simulink model "TSR_Scenario_002_cs"  (R2014b)
settings: Solver=ode5  SolverMode=SingleTasking  StartTime=0.0  StopTime=inf  FixedStep=1/100  RelTol=1e-3
PreLoadFcn:
  | mbxruntime.callbacks.PreLoadFcn(bdroot);
  | check_NUTS_defined;
  | 
  | assignin('base',['model_closed_' bdroot],false);
  | 
  | addpath('../includes_TSR/includes_TSR');
  | 
  | switch version('-release')
  | case {'2010a', '2010b', '2011a'}
  | addpath('../includes_TSR/ML2010b');
  | otherwise
  | addpath('../includes_TSR/ML2011b');
  | end
PostLoadFcn:
  | mbxruntime.callbacks.PostLoadFcn(bdroot);
InitFcn:
  | mbxruntime.callbacks.InitFcn(bdroot);;
  | 
  | addpath('..\includes_TSR');
StartFcn:
  | mbxruntime.callbacks.StartFcn(bdroot);
StopFcn:
  | mbxruntime.callbacks.StopFcn(bdroot);
model workspace: external: MAT-File .\TSR_Scenario_002_cs_hws.mat (data not in the file)
undefined symbols (not defined in the file or in its folder): InitImageOutputDir, mbxruntime, OrientationPitch, OrientationRoll, PositionX, PositionY, PositionZ, tabledata, warningInitialVelocity, x0
undefined symbols (not defined in the file): SteeringColumn, SteeringWheel, TSR_Scenario_002_cs_003e47b1b59594b6, TSR_Scenario_002_cs_023e87a31011dc74, TSR_Scenario_002_cs_048cb8409c90d9c6, TSR_Scenario_002_cs_106a0284aafa53e6, TSR_Scenario_002_cs_195b368d22a7f172, TSR_Scenario_002_cs_1e339fa5d680f213, TSR_Scenario_002_cs_26196a9fb104f950, TSR_Scenario_002_cs_261a709f6f453598, TSR_Scenario_002_cs_2ac3337370d0049d, TSR_Scenario_002_cs_2dc51e6a68b01b00, TSR_Scenario_002_cs_3460ff54d38ab2e2, TSR_Scenario_002_cs_42ea7d6e56bd6005, TSR_Scenario_002_cs_4dd419d6d2b56fc2, TSR_Scenario_002_cs_5316a21de09dff2f, TSR_Scenario_002_cs_538caacf3455966d, TSR_Scenario_002_cs_5b2cfdbcfc80811f, TSR_Scenario_002_cs_5ce0eafbb7a2dce7, TSR_Scenario_002_cs_62cdbf45c6f8824a, TSR_Scenario_002_cs_6bebc368eedff0bc, TSR_Scenario_002_cs_6d26481da4ed7e29, TSR_Scenario_002_cs_70c7e369ce6550e0, TSR_Scenario_002_cs_7a63051a1f311451, TSR_Scenario_002_cs_7d7dc8405f613c6d, TSR_Scenario_002_cs_7f65e296173485e8, TSR_Scenario_002_cs_87183cf6ff7bb4b6, TSR_Scenario_002_cs_8921b0da7ab80865, TSR_Scenario_002_cs_9495ce3a76763d1f, TSR_Scenario_002_cs_a679806a2fdc8099, TSR_Scenario_002_cs_Actros_1860_1_Path_pathUniqueID, TSR_Scenario_002_cs_Actros_2541_1_Path_pathUniqueID, TSR_Scenario_002_cs_Actros_2541_3_Path_pathUniqueID, TSR_Scenario_002_cs_Actros_2541_4_Path_pathUniqueID, TSR_Scenario_002_cs_adf24c93a9de8a4e, TSR_Scenario_002_cs_Audi_A8_1_Dynamics_Simple_initialPitch, TSR_Scenario_002_cs_Audi_A8_1_Dynamics_Simple_initialRoll, TSR_Scenario_002_cs_Audi_A8_1_Dynamics_Simple_initialX, TSR_Scenario_002_cs_Audi_A8_1_Dynamics_Simple_initialY, TSR_Scenario_002_cs_Audi_A8_1_Dynamics_Simple_initialYaw, TSR_Scenario_002_cs_Audi_A8_1_Dynamics_Simple_initialZ, TSR_Scenario_002_cs_b136c6ccb55f77db, TSR_Scenario_002_cs_ba4f809714c282b7, TSR_Scenario_002_cs_BMW_X5_1_Path_pathUniqueID, TSR_Scenario_002_cs_BMW_X5_1_SpeedProfile_speedProfileUniqueID, TSR_Scenario_002_cs_BMW_X5_2_Path_pathUniqueID, TSR_Scenario_002_cs_BMW_X5_2_SpeedProfile_speedProfileUniqueID, TSR_Scenario_002_cs_Citroen_C3_1_Path_pathUniqueID, TSR_Scenario_002_cs_Citroen_C3_2_Path_pathUniqueID, TSR_Scenario_002_cs_d8f275339b7082cf, TSR_Scenario_002_cs_Daf_95_1_Path_pathUniqueID, TSR_Scenario_002_cs_Daf_95_1_SpeedProfile_speedProfileUniqueID, TSR_Scenario_002_cs_dc019741510ce2f2, TSR_Scenario_002_cs_fdbc8aabe460b27c, TSR_Scenario_002_cs_Fiat_Bravo_1_Path_pathUniqueID, TSR_Scenario_002_cs_Ford_Fiesta_1_Path_pathUniqueID, TSR_Scenario_002_cs_Honda_Pan_European_1_Path_pathUniqueID, TSR_Scenario_002_cs_Mazda_RX8_1_Path_pathUniqueID, TSR_Scenario_002_cs_Nissan_Cabstar_1_Path_pathUniqueID, TSR_Scenario_002_cs_Nissan_Cabstar_2_Path_pathUniqueID ... (+9)
libraries: simulink_extras x82, simulink x23, PreScanSimulinkLibrary x11
(part 20 of 39)

== system TSR_Scenario_002_cs/Fiat_Bravo_1/SELF_Demux ==
  SELF : Inport  OutDataTypeStr=Bus: PRESCAN_SELFSENSORDATA
  Bus Selector : BusSelector  OutputSignals=PositionX,PositionY,PositionZ,OrientationRoll,OrientationPitch,OrientationYaw,Velocity,Yaw_rate,Lat,Long,Alt
  Demux2 : Demux  Outputs=3
  Gain : Gain  Gain=180/pi
  Gain1 : Gain  Gain=180/pi
  Vector Concatenate1 : Concatenate  NumInputs=3
  compas converter : Subsystem
  x [m] : Outport
  y [m] : Outport  Port=2
  z [m] : Outport  Port=3
  rotx [deg] : Outport  Port=4
  roty [deg] : Outport  Port=5
  rotz [deg] : Outport  Port=6
  GPS lat [deg] : Outport  Port=7
  GPS long [deg] : Outport  Port=8
  GPS alt [m] : Outport  Port=9
  velocity [m/s] : Outport  Port=10
  heading [deg] : Outport  Port=11
  yaw rate [deg/s] : Outport  Port=12
  wires:
  Bus Selector/11 -> GPS alt [m]/1  "<Alt>"
  Bus Selector/10 -> GPS long [deg]/1  "<Long>"
  Bus Selector/9 -> GPS lat [deg]/1  "<Lat>"
  Bus Selector/8 -> Gain1/1  "<Yaw_rate>"
  Bus Selector/7 -> velocity [m/s]/1  "<Velocity>"
  Bus Selector/6 -> compas converter/1(rotz [rad]), Vector Concatenate1/3  "<OrientationYaw>"
  Bus Selector/5 -> Vector Concatenate1/2  "<OrientationPitch>"
  Bus Selector/4 -> Vector Concatenate1/1  "<OrientationRoll>"
  Vector Concatenate1/1 -> Gain/1
  Bus Selector/3 -> z [m]/1  "<PositionZ>"
  Bus Selector/2 -> y [m]/1  "<PositionY>"
  Bus Selector/1 -> x [m]/1  "<PositionX>"
  SELF/1 -> Bus Selector/1
  Gain/1 -> Demux2/1
  Demux2/1 -> rotx [deg]/1
  Demux2/2 -> roty [deg]/1
  Demux2/3 -> rotz [deg]/1
  compas converter/1(heading [deg]) -> heading [deg]/1
  Gain1/1 -> yaw rate [deg/s]/1

== system TSR_Scenario_002_cs/Fiat_Bravo_1/SteeringColumn_pivot_Mux ==
  X [m] : Inport
  Y [m] : Inport  Port=2
  Z [m] : Inport  Port=3
  Roll [rad] : Inport  Port=4
  Pitch [rad] : Inport  Port=5
  Yaw [rad] : Inport  Port=6
  Bus Creator : BusCreator  Inputs=3  OutDataTypeStr=Bus: PRESCAN_XYZ_DATA
  Bus Creator1 : BusCreator  Inputs=3  OutDataTypeStr=Bus: PRESCAN_RPY_DATA
  Bus Creator2 : BusCreator  Inputs=2  OutDataTypeStr=Bus: PRESCAN_POSE_DATA
  Joint : Outport
  wires:
  Yaw [rad]/1 -> Bus Creator1/3  "Yaw"
  Bus Creator1/1 -> Bus Creator2/2  "ORIENTATION"
  Bus Creator/1 -> Bus Creator2/1  "POSITION"
  X [m]/1 -> Bus Creator/1  "X"
  Y [m]/1 -> Bus Creator/2  "Y"
  Z [m]/1 -> Bus Creator/3  "Z"
  Bus Creator2/1 -> Joint/1
  Roll [rad]/1 -> Bus Creator1/1  "Roll"
  Pitch [rad]/1 -> Bus Creator1/2  "Pitch"

== system TSR_Scenario_002_cs/Fiat_Bravo_1/SteeringWheel_pivot_Mux ==
  X [m] : Inport
  Y [m] : Inport  Port=2
  Z [m] : Inport  Port=3
  Roll [rad] : Inport  Port=4
  Pitch [rad] : Inport  Port=5
  Yaw [rad] : Inport  Port=6
  Bus Creator : BusCreator  Inputs=3  OutDataTypeStr=Bus: PRESCAN_XYZ_DATA
  Bus Creator1 : BusCreator  Inputs=3  OutDataTypeStr=Bus: PRESCAN_RPY_DATA
  Bus Creator2 : BusCreator  Inputs=2  OutDataTypeStr=Bus: PRESCAN_POSE_DATA
  Joint : Outport
  wires:
  Yaw [rad]/1 -> Bus Creator1/3  "Yaw"
  Bus Creator1/1 -> Bus Creator2/2  "ORIENTATION"
  Bus Creator/1 -> Bus Creator2/1  "POSITION"
  X [m]/1 -> Bus Creator/1  "X"
  Y [m]/1 -> Bus Creator/2  "Y"
  Z [m]/1 -> Bus Creator/3  "Z"
  Bus Creator2/1 -> Joint/1
  Roll [rad]/1 -> Bus Creator1/1  "Roll"
  Pitch [rad]/1 -> Bus Creator1/2  "Pitch"

== system TSR_Scenario_002_cs/Fiat_Bravo_1/WheelDisplacement_Mux ==
  Steering Angle Front [rad] : Inport  Tag=inport/JointGroup  SampleTime=1/100  BusOutputAsStruct=on
  Steering Angle Rear [rad] : Inport  Tag=inport/JointGroup  Port=2  SampleTime=1/100  BusOutputAsStruct=on
  Rotation [rad] : Inport  Tag=inport/JointGroup  Port=3  SampleTime=1/100  BusOutputAsStruct=on
  zDisp FL [m] : Inport  Tag=inport/JointGroup  Port=4  SampleTime=1/100  BusOutputAsStruct=on
  zDisp FR [m] : Inport  Tag=inport/JointGroup  Port=5  SampleTime=1/100  BusOutputAsStruct=on
  zDisp RL [m] : Inport  Tag=inport/JointGroup  Port=6  SampleTime=1/100  BusOutputAsStruct=on
  zDisp RR [m] : Inport  Tag=inport/JointGroup  Port=7  SampleTime=1/100  BusOutputAsStruct=on
  Ground_{1..12} (12 alike) : Ground
  WheelL0_Mux : Subsystem  Tag=mux/Joint  mask(PreScan Mux Block){DisplayName=WheelL0}
      mask prompts: DisplayName "Display Name"
      mask help:
      | This block simulates a generic joint used for generic models. This joint can be enabled/disabled from the GUI.
      |
      | For more information, please click Help.
      settings: DeleteFcn=PreScanBlockDeleteFcn;
      mask Help: eval('openHelp(254)')
  WheelL1_Mux : Subsystem  Tag=mux/Joint  mask(PreScan Mux Block){DisplayName=WheelL1}
      mask prompts: DisplayName "Display Name"
      mask help:
      | This block simulates a generic joint used for generic models. This joint can be enabled/disabled from the GUI.
      |
      | For more information, please click Help.
      settings: DeleteFcn=PreScanBlockDeleteFcn;
      mask Help: eval('openHelp(254)')
  WheelR0_Mux : Subsystem  Tag=mux/Joint  mask(PreScan Mux Block){DisplayName=WheelR0}
      mask prompts: DisplayName "Display Name"
      mask help:
      | This block simulates a generic joint used for generic models. This joint can be enabled/disabled from the GUI.
      |
      | For more information, please click Help.
      settings: DeleteFcn=PreScanBlockDeleteFcn;
      mask Help: eval('openHelp(254)')
  WheelR1_Mux : Subsystem  Tag=mux/Joint  mask(PreScan Mux Block){DisplayName=WheelR1}
      mask prompts: DisplayName "Display Name"
      mask help:
      | This block simulates a generic joint used for generic models. This joint can be enabled/disabled from the GUI.
      |
      | For more information, please click Help.
      settings: DeleteFcn=PreScanBlockDeleteFcn;
      mask Help: eval('openHelp(254)')
  WheelL0_Fiat_Bravo_1 : Outport  Tag=outport/JointActuator  OutDataTypeStr=Bus: PRESCAN_POSE_DATA  SampleTime=1/100
  WheelL1_Fiat_Bravo_1 : Outport  Tag=outport/JointActuator  Port=2  OutDataTypeStr=Bus: PRESCAN_POSE_DATA  SampleTime=1/100
  WheelR0_Fiat_Bravo_1 : Outport  Tag=outport/JointActuator  Port=3  OutDataTypeStr=Bus: PRESCAN_POSE_DATA  SampleTime=1/100
  WheelR1_Fiat_Bravo_1 : Outport  Tag=outport/JointActuator  Port=4  OutDataTypeStr=Bus: PRESCAN_POSE_DATA  SampleTime=1/100
  wires:
  WheelL0_Mux/1(Joint) -> WheelL0_Fiat_Bravo_1/1
  WheelL1_Mux/1(Joint) -> WheelL1_Fiat_Bravo_1/1
  WheelR0_Mux/1(Joint) -> WheelR0_Fiat_Bravo_1/1
  WheelR1_Mux/1(Joint) -> WheelR1_Fiat_Bravo_1/1
  Steering Angle Front [rad]/1 -> WheelR0_Mux/6(Yaw [rad]), WheelL0_Mux/6(Yaw [rad])
  Steering Angle Rear [rad]/1 -> WheelR1_Mux/6(Yaw [rad]), WheelL1_Mux/6(Yaw [rad])
  Rotation [rad]/1 -> WheelR0_Mux/5(Pitch [rad]), WheelL0_Mux/5(Pitch [rad]), WheelR1_Mux/5(Pitch [rad]), WheelL1_Mux/5(Pitch [rad])
  zDisp FL [m]/1 -> WheelL0_Mux/3(Z [m])
  zDisp FR [m]/1 -> WheelR0_Mux/3(Z [m])
  zDisp RL [m]/1 -> WheelL1_Mux/3(Z [m])
  zDisp RR [m]/1 -> WheelR1_Mux/3(Z [m])
  Ground_1/1 -> WheelL0_Mux/1(X [m])
  Ground_2/1 -> WheelL0_Mux/2(Y [m])
  Ground_3/1 -> WheelL0_Mux/4(Roll [rad])
  Ground_4/1 -> WheelL1_Mux/1(X [m])
  Ground_5/1 -> WheelL1_Mux/2(Y [m])
  Ground_6/1 -> WheelL1_Mux/4(Roll [rad])
  Ground_7/1 -> WheelR0_Mux/1(X [m])
  Ground_8/1 -> WheelR0_Mux/2(Y [m])
  Ground_9/1 -> WheelR0_Mux/4(Roll [rad])
  Ground_10/1 -> WheelR1_Mux/1(X [m])
  Ground_11/1 -> WheelR1_Mux/2(Y [m])
  Ground_12/1 -> WheelR1_Mux/4(Roll [rad])

== system TSR_Scenario_002_cs/Ford_Fiesta_1/SELF_Demux ==
  SELF : Inport  OutDataTypeStr=Bus: PRESCAN_SELFSENSORDATA
  Bus Selector : BusSelector  OutputSignals=PositionX,PositionY,PositionZ,OrientationRoll,OrientationPitch,OrientationYaw,Velocity,Yaw_rate,Lat,Long,Alt
  Demux2 : Demux  Outputs=3
  Gain : Gain  Gain=180/pi
  Gain1 : Gain  Gain=180/pi
  Vector Concatenate1 : Concatenate  NumInputs=3
  compas converter : Subsystem
  x [m] : Outport
  y [m] : Outport  Port=2
  z [m] : Outport  Port=3
  rotx [deg] : Outport  Port=4
  roty [deg] : Outport  Port=5
  rotz [deg] : Outport  Port=6
  GPS lat [deg] : Outport  Port=7
  GPS long [deg] : Outport  Port=8
  GPS alt [m] : Outport  Port=9
  velocity [m/s] : Outport  Port=10
  heading [deg] : Outport  Port=11
  yaw rate [deg/s] : Outport  Port=12
  wires:
  Bus Selector/11 -> GPS alt [m]/1  "<Alt>"
  Bus Selector/10 -> GPS long [deg]/1  "<Long>"
  Bus Selector/9 -> GPS lat [deg]/1  "<Lat>"
  Bus Selector/8 -> Gain1/1  "<Yaw_rate>"
  Bus Selector/7 -> velocity [m/s]/1  "<Velocity>"
  Bus Selector/6 -> compas converter/1(rotz [rad]), Vector Concatenate1/3  "<OrientationYaw>"
  Bus Selector/5 -> Vector Concatenate1/2  "<OrientationPitch>"
  Bus Selector/4 -> Vector Concatenate1/1  "<OrientationRoll>"
  Vector Concatenate1/1 -> Gain/1
  Bus Selector/3 -> z [m]/1  "<PositionZ>"
  Bus Selector/2 -> y [m]/1  "<PositionY>"
  Bus Selector/1 -> x [m]/1  "<PositionX>"
  SELF/1 -> Bus Selector/1
  Gain/1 -> Demux2/1
  Demux2/1 -> rotx [deg]/1
  Demux2/2 -> roty [deg]/1
  Demux2/3 -> rotz [deg]/1
  compas converter/1(heading [deg]) -> heading [deg]/1
  Gain1/1 -> yaw rate [deg/s]/1

== system TSR_Scenario_002_cs/HighwayOverhang_1/VISUMatrixSignLights_Mux ==
  MatrixSign_1 : Inport  Tag=inport/MatrixSign_1  PortDimensions=4  SampleTime=1/100  BusOutputAsStruct=on
  MatrixSign_43 : Inport  Tag=inport/MatrixSign_43  Port=2  PortDimensions=4  SampleTime=1/100  BusOutputAsStruct=on
  MuxVisuLights : Mux  Inputs=2
  VISUMatrixSignLights_HighwayOverhang_1 : Outport  Tag=outport/VisuMatrixSignLights  SampleTime=1/100
  wires:
  MuxVisuLights/1 -> VISUMatrixSignLights_HighwayOverhang_1/1
  MatrixSign_1/1 -> MuxVisuLights/1
  MatrixSign_43/1 -> MuxVisuLights/2

== system TSR_Scenario_002_cs/HighwayOverhang_1/VISUMatrixSign_Mux ==
  MatrixSign_1 : Inport
  MatrixSign_43 : Inport  Port=2
  MatrixSign_1_Conversion : DataTypeConversion
  MatrixSign_1_InitialResource : Constant  Value=17
  MatrixSign_1_Switch : Switch  Criteria=u2 ~= 0
  MatrixSign_43_Conversion : DataTypeConversion
  MatrixSign_43_InitialResource : Constant  Value=17
  MatrixSign_43_Switch : Switch  Criteria=u2 ~= 0
  SubMuxMatrixSign : Mux  Inputs=2
  MatrixSigns : Outport
  wires:
  SubMuxMatrixSign/1 -> MatrixSigns/1
  MatrixSign_1/1 -> MatrixSign_1_Switch/1, MatrixSign_1_Switch/2
  MatrixSign_1_InitialResource/1 -> MatrixSign_1_Switch/3
  MatrixSign_1_Switch/1 -> MatrixSign_1_Conversion/1
  MatrixSign_1_Conversion/1 -> SubMuxMatrixSign/1
  MatrixSign_43/1 -> MatrixSign_43_Switch/1, MatrixSign_43_Switch/2
  MatrixSign_43_InitialResource/1 -> MatrixSign_43_Switch/3
  MatrixSign_43_Switch/1 -> MatrixSign_43_Conversion/1
  MatrixSign_43_Conversion/1 -> SubMuxMatrixSign/2

== system TSR_Scenario_002_cs/HighwayOverhang_10/VISUMatrixSignLights_Mux ==
  MatrixSign_17 : Inport  Tag=inport/MatrixSign_17  PortDimensions=4  SampleTime=1/100  BusOutputAsStruct=on
  MatrixSign_18 : Inport  Tag=inport/MatrixSign_18  Port=2  PortDimensions=4  SampleTime=1/100  BusOutputAsStruct=on
  MuxVisuLights : Mux  Inputs=2
  VISUMatrixSignLights_HighwayOverhang_10 : Outport  Tag=outport/VisuMatrixSignLights  SampleTime=1/100
  wires:
  MuxVisuLights/1 -> VISUMatrixSignLights_HighwayOverhang_10/1
  MatrixSign_17/1 -> MuxVisuLights/1
  MatrixSign_18/1 -> MuxVisuLights/2

== system TSR_Scenario_002_cs/HighwayOverhang_10/VISUMatrixSign_Mux ==
  MatrixSign_17 : Inport
  MatrixSign_18 : Inport  Port=2
  MatrixSign_17_Conversion : DataTypeConversion
  MatrixSign_17_InitialResource : Constant
  MatrixSign_17_Switch : Switch  Criteria=u2 ~= 0
  MatrixSign_18_Conversion : DataTypeConversion
  MatrixSign_18_InitialResource : Constant
  MatrixSign_18_Switch : Switch  Criteria=u2 ~= 0
  SubMuxMatrixSign : Mux  Inputs=2
  MatrixSigns : Outport
  wires:
  SubMuxMatrixSign/1 -> MatrixSigns/1
  MatrixSign_17/1 -> MatrixSign_17_Switch/1, MatrixSign_17_Switch/2
  MatrixSign_17_InitialResource/1 -> MatrixSign_17_Switch/3
  MatrixSign_17_Switch/1 -> MatrixSign_17_Conversion/1
  MatrixSign_17_Conversion/1 -> SubMuxMatrixSign/1
  MatrixSign_18/1 -> MatrixSign_18_Switch/1, MatrixSign_18_Switch/2
  MatrixSign_18_InitialResource/1 -> MatrixSign_18_Switch/3
  MatrixSign_18_Switch/1 -> MatrixSign_18_Conversion/1
  MatrixSign_18_Conversion/1 -> SubMuxMatrixSign/2

== system TSR_Scenario_002_cs/HighwayOverhang_11/VISUMatrixSignLights_Mux ==
  MatrixSign_10 : Inport  Tag=inport/MatrixSign_10  PortDimensions=4  SampleTime=1/100  BusOutputAsStruct=on
  MatrixSign_49 : Inport  Tag=inport/MatrixSign_49  Port=2  PortDimensions=4  SampleTime=1/100  BusOutputAsStruct=on
  MuxVisuLights : Mux  Inputs=2
  VISUMatrixSignLights_HighwayOverhang_11 : Outport  Tag=outport/VisuMatrixSignLights  SampleTime=1/100
  wires:
  MuxVisuLights/1 -> VISUMatrixSignLights_HighwayOverhang_11/1
  MatrixSign_10/1 -> MuxVisuLights/1
  MatrixSign_49/1 -> MuxVisuLights/2

== system TSR_Scenario_002_cs/HighwayOverhang_11/VISUMatrixSign_Mux ==
  MatrixSign_10 : Inport
  MatrixSign_49 : Inport  Port=2
  MatrixSign_10_Conversion : DataTypeConversion
  MatrixSign_10_InitialResource : Constant  Value=11
  MatrixSign_10_Switch : Switch  Criteria=u2 ~= 0
  MatrixSign_49_Conversion : DataTypeConversion
  MatrixSign_49_InitialResource : Constant  Value=11
  MatrixSign_49_Switch : Switch  Criteria=u2 ~= 0
  SubMuxMatrixSign : Mux  Inputs=2
  MatrixSigns : Outport
  wires:
  SubMuxMatrixSign/1 -> MatrixSigns/1
  MatrixSign_10/1 -> MatrixSign_10_Switch/1, MatrixSign_10_Switch/2
  MatrixSign_10_InitialResource/1 -> MatrixSign_10_Switch/3
  MatrixSign_10_Switch/1 -> MatrixSign_10_Conversion/1
  MatrixSign_10_Conversion/1 -> SubMuxMatrixSign/1
  MatrixSign_49/1 -> MatrixSign_49_Switch/1, MatrixSign_49_Switch/2
  MatrixSign_49_InitialResource/1 -> MatrixSign_49_Switch/3
  MatrixSign_49_Switch/1 -> MatrixSign_49_Conversion/1
  MatrixSign_49_Conversion/1 -> SubMuxMatrixSign/2

== system TSR_Scenario_002_cs/HighwayOverhang_12/VISUMatrixSignLights_Mux ==
  MatrixSign_21 : Inport  Tag=inport/MatrixSign_21  PortDimensions=4  SampleTime=1/100  BusOutputAsStruct=on
  MatrixSign_22 : Inport  Tag=inport/MatrixSign_22  Port=2  PortDimensions=4  SampleTime=1/100  BusOutputAsStruct=on
  MuxVisuLights : Mux  Inputs=2
  VISUMatrixSignLights_HighwayOverhang_12 : Outport  Tag=outport/VisuMatrixSignLights  SampleTime=1/100
  wires:
  MuxVisuLights/1 -> VISUMatrixSignLights_HighwayOverhang_12/1
  MatrixSign_21/1 -> MuxVisuLights/1
  MatrixSign_22/1 -> MuxVisuLights/2

== system TSR_Scenario_002_cs/HighwayOverhang_12/VISUMatrixSign_Mux ==
  MatrixSign_21 : Inport
  MatrixSign_22 : Inport  Port=2
  MatrixSign_21_Conversion : DataTypeConversion
  MatrixSign_21_InitialResource : Constant
  MatrixSign_21_Switch : Switch  Criteria=u2 ~= 0
  MatrixSign_22_Conversion : DataTypeConversion
  MatrixSign_22_InitialResource : Constant
  MatrixSign_22_Switch : Switch  Criteria=u2 ~= 0
  SubMuxMatrixSign : Mux  Inputs=2
  MatrixSigns : Outport
  wires:
  SubMuxMatrixSign/1 -> MatrixSigns/1
  MatrixSign_21/1 -> MatrixSign_21_Switch/1, MatrixSign_21_Switch/2
  MatrixSign_21_InitialResource/1 -> MatrixSign_21_Switch/3
  MatrixSign_21_Switch/1 -> MatrixSign_21_Conversion/1
  MatrixSign_21_Conversion/1 -> SubMuxMatrixSign/1
  MatrixSign_22/1 -> MatrixSign_22_Switch/1, MatrixSign_22_Switch/2
  MatrixSign_22_InitialResource/1 -> MatrixSign_22_Switch/3
  MatrixSign_22_Switch/1 -> MatrixSign_22_Conversion/1
  MatrixSign_22_Conversion/1 -> SubMuxMatrixSign/2

== system TSR_Scenario_002_cs/HighwayOverhang_13/VISUMatrixSignLights_Mux ==
  MatrixSign_3 : Inport  Tag=inport/MatrixSign_3  PortDimensions=4  SampleTime=1/100  BusOutputAsStruct=on
  MatrixSign_44 : Inport  Tag=inport/MatrixSign_44  Port=2  PortDimensions=4  SampleTime=1/100  BusOutputAsStruct=on
  MuxVisuLights : Mux  Inputs=2
  VISUMatrixSignLights_HighwayOverhang_13 : Outport  Tag=outport/VisuMatrixSignLights  SampleTime=1/100
  wires:
  MuxVisuLights/1 -> VISUMatrixSignLights_HighwayOverhang_13/1
  MatrixSign_3/1 -> MuxVisuLights/1
  MatrixSign_44/1 -> MuxVisuLights/2

== system TSR_Scenario_002_cs/HighwayOverhang_13/VISUMatrixSign_Mux ==
  MatrixSign_3 : Inport
  MatrixSign_44 : Inport  Port=2
  MatrixSign_3_Conversion : DataTypeConversion
  MatrixSign_3_InitialResource : Constant  Value=16
  MatrixSign_3_Switch : Switch  Criteria=u2 ~= 0
  MatrixSign_44_Conversion : DataTypeConversion
  MatrixSign_44_InitialResource : Constant  Value=16
  MatrixSign_44_Switch : Switch  Criteria=u2 ~= 0
  SubMuxMatrixSign : Mux  Inputs=2
  MatrixSigns : Outport
  wires:
  SubMuxMatrixSign/1 -> MatrixSigns/1
  MatrixSign_3/1 -> MatrixSign_3_Switch/1, MatrixSign_3_Switch/2
  MatrixSign_3_InitialResource/1 -> MatrixSign_3_Switch/3
  MatrixSign_3_Switch/1 -> MatrixSign_3_Conversion/1
  MatrixSign_3_Conversion/1 -> SubMuxMatrixSign/1
  MatrixSign_44/1 -> MatrixSign_44_Switch/1, MatrixSign_44_Switch/2
  MatrixSign_44_InitialResource/1 -> MatrixSign_44_Switch/3
  MatrixSign_44_Switch/1 -> MatrixSign_44_Conversion/1
  MatrixSign_44_Conversion/1 -> SubMuxMatrixSign/2

== system TSR_Scenario_002_cs/HighwayOverhang_14/VISUMatrixSignLights_Mux ==
  MatrixSign_27 : Inport  Tag=inport/MatrixSign_27  PortDimensions=4  SampleTime=1/100  BusOutputAsStruct=on
  MatrixSign_28 : Inport  Tag=inport/MatrixSign_28  Port=2  PortDimensions=4  SampleTime=1/100  BusOutputAsStruct=on
  MuxVisuLights : Mux  Inputs=2
  VISUMatrixSignLights_HighwayOverhang_14 : Outport  Tag=outport/VisuMatrixSignLights  SampleTime=1/100
  wires:
  MuxVisuLights/1 -> VISUMatrixSignLights_HighwayOverhang_14/1
  MatrixSign_27/1 -> MuxVisuLights/1
  MatrixSign_28/1 -> MuxVisuLights/2

== system TSR_Scenario_002_cs/HighwayOverhang_14/VISUMatrixSign_Mux ==
  MatrixSign_27 : Inport
  MatrixSign_28 : Inport  Port=2
  MatrixSign_27_Conversion : DataTypeConversion
  MatrixSign_27_InitialResource : Constant
  MatrixSign_27_Switch : Switch  Criteria=u2 ~= 0
  MatrixSign_28_Conversion : DataTypeConversion
  MatrixSign_28_InitialResource : Constant
  MatrixSign_28_Switch : Switch  Criteria=u2 ~= 0
  SubMuxMatrixSign : Mux  Inputs=2
  MatrixSigns : Outport
  wires:
  SubMuxMatrixSign/1 -> MatrixSigns/1
  MatrixSign_27/1 -> MatrixSign_27_Switch/1, MatrixSign_27_Switch/2
  MatrixSign_27_InitialResource/1 -> MatrixSign_27_Switch/3
  MatrixSign_27_Switch/1 -> MatrixSign_27_Conversion/1
  MatrixSign_27_Conversion/1 -> SubMuxMatrixSign/1
  MatrixSign_28/1 -> MatrixSign_28_Switch/1, MatrixSign_28_Switch/2
  MatrixSign_28_InitialResource/1 -> MatrixSign_28_Switch/3
  MatrixSign_28_Switch/1 -> MatrixSign_28_Conversion/1
  MatrixSign_28_Conversion/1 -> SubMuxMatrixSign/2

== system TSR_Scenario_002_cs/HighwayOverhang_15/VISUMatrixSignLights_Mux ==
  MatrixSign_46 : Inport  Tag=inport/MatrixSign_46  PortDimensions=4  SampleTime=1/100  BusOutputAsStruct=on
  MatrixSign_5 : Inport  Tag=inport/MatrixSign_5  Port=2  PortDimensions=4  SampleTime=1/100  BusOutputAsStruct=on
  MuxVisuLights : Mux  Inputs=2
  VISUMatrixSignLights_HighwayOverhang_15 : Outport  Tag=outport/VisuMatrixSignLights  SampleTime=1/100
  wires:
  MuxVisuLights/1 -> VISUMatrixSignLights_HighwayOverhang_15/1
  MatrixSign_46/1 -> MuxVisuLights/1
  MatrixSign_5/1 -> MuxVisuLights/2

== system TSR_Scenario_002_cs/HighwayOverhang_15/VISUMatrixSign_Mux ==
  MatrixSign_5 : Inport
  MatrixSign_46 : Inport  Port=2
  MatrixSign_46_Conversion : DataTypeConversion
  MatrixSign_46_InitialResource : Constant  Value=14
  MatrixSign_46_Switch : Switch  Criteria=u2 ~= 0
  MatrixSign_5_Conversion : DataTypeConversion
  MatrixSign_5_InitialResource : Constant  Value=14
  MatrixSign_5_Switch : Switch  Criteria=u2 ~= 0
  SubMuxMatrixSign : Mux  Inputs=2
  MatrixSigns : Outport
  wires:
  SubMuxMatrixSign/1 -> MatrixSigns/1
  MatrixSign_5/1 -> MatrixSign_5_Switch/1, MatrixSign_5_Switch/2
  MatrixSign_5_InitialResource/1 -> MatrixSign_5_Switch/3
  MatrixSign_5_Switch/1 -> MatrixSign_5_Conversion/1
  MatrixSign_5_Conversion/1 -> SubMuxMatrixSign/1
  MatrixSign_46/1 -> MatrixSign_46_Switch/1, MatrixSign_46_Switch/2
  MatrixSign_46_InitialResource/1 -> MatrixSign_46_Switch/3
  MatrixSign_46_Switch/1 -> MatrixSign_46_Conversion/1
  MatrixSign_46_Conversion/1 -> SubMuxMatrixSign/2

== system TSR_Scenario_002_cs/HighwayOverhang_16/VISUMatrixSignLights_Mux ==
  MatrixSign_29 : Inport  Tag=inport/MatrixSign_29  PortDimensions=4  SampleTime=1/100  BusOutputAsStruct=on
  MatrixSign_30 : Inport  Tag=inport/MatrixSign_30  Port=2  PortDimensions=4  SampleTime=1/100  BusOutputAsStruct=on
  MuxVisuLights : Mux  Inputs=2
  VISUMatrixSignLights_HighwayOverhang_16 : Outport  Tag=outport/VisuMatrixSignLights  SampleTime=1/100
  wires:
  MuxVisuLights/1 -> VISUMatrixSignLights_HighwayOverhang_16/1
  MatrixSign_29/1 -> MuxVisuLights/1
  MatrixSign_30/1 -> MuxVisuLights/2

== system TSR_Scenario_002_cs/HighwayOverhang_16/VISUMatrixSign_Mux ==
  MatrixSign_29 : Inport
  MatrixSign_30 : Inport  Port=2
  MatrixSign_29_Conversion : DataTypeConversion
  MatrixSign_29_InitialResource : Constant
  MatrixSign_29_Switch : Switch  Criteria=u2 ~= 0
  MatrixSign_30_Conversion : DataTypeConversion
  MatrixSign_30_InitialResource : Constant
  MatrixSign_30_Switch : Switch  Criteria=u2 ~= 0
  SubMuxMatrixSign : Mux  Inputs=2
  MatrixSigns : Outport
  wires:
  SubMuxMatrixSign/1 -> MatrixSigns/1
  MatrixSign_29/1 -> MatrixSign_29_Switch/1, MatrixSign_29_Switch/2
  MatrixSign_29_InitialResource/1 -> MatrixSign_29_Switch/3
  MatrixSign_29_Switch/1 -> MatrixSign_29_Conversion/1
  MatrixSign_29_Conversion/1 -> SubMuxMatrixSign/1
  MatrixSign_30/1 -> MatrixSign_30_Switch/1, MatrixSign_30_Switch/2
  MatrixSign_30_InitialResource/1 -> MatrixSign_30_Switch/3
  MatrixSign_30_Switch/1 -> MatrixSign_30_Conversion/1
  MatrixSign_30_Conversion/1 -> SubMuxMatrixSign/2

== system TSR_Scenario_002_cs/HighwayOverhang_17/VISUMatrixSignLights_Mux ==
  MatrixSign_51 : Inport  Tag=inport/MatrixSign_51  PortDimensions=4  SampleTime=1/100  BusOutputAsStruct=on
  MatrixSign_7 : Inport  Tag=inport/MatrixSign_7  Port=2  PortDimensions=4  SampleTime=1/100  BusOutputAsStruct=on
  MuxVisuLights : Mux  Inputs=2
  VISUMatrixSignLights_HighwayOverhang_17 : Outport  Tag=outport/VisuMatrixSignLights  SampleTime=1/100
  wires:
  MuxVisuLights/1 -> VISUMatrixSignLights_HighwayOverhang_17/1
  MatrixSign_51/1 -> MuxVisuLights/1
  MatrixSign_7/1 -> MuxVisuLights/2

== system TSR_Scenario_002_cs/HighwayOverhang_17/VISUMatrixSign_Mux ==
  MatrixSign_7 : Inport
  MatrixSign_51 : Inport  Port=2
  MatrixSign_51_Conversion : DataTypeConversion
  MatrixSign_51_InitialResource : Constant  Value=9
  MatrixSign_51_Switch : Switch  Criteria=u2 ~= 0
  MatrixSign_7_Conversion : DataTypeConversion
  MatrixSign_7_InitialResource : Constant  Value=9
  MatrixSign_7_Switch : Switch  Criteria=u2 ~= 0
  SubMuxMatrixSign : Mux  Inputs=2
  MatrixSigns : Outport
  wires:
  SubMuxMatrixSign/1 -> MatrixSigns/1
  MatrixSign_7/1 -> MatrixSign_7_Switch/1, MatrixSign_7_Switch/2
  MatrixSign_7_InitialResource/1 -> MatrixSign_7_Switch/3
  MatrixSign_7_Switch/1 -> MatrixSign_7_Conversion/1
  MatrixSign_7_Conversion/1 -> SubMuxMatrixSign/1
  MatrixSign_51/1 -> MatrixSign_51_Switch/1, MatrixSign_51_Switch/2
  MatrixSign_51_InitialResource/1 -> MatrixSign_51_Switch/3
  MatrixSign_51_Switch/1 -> MatrixSign_51_Conversion/1
  MatrixSign_51_Conversion/1 -> SubMuxMatrixSign/2

== system TSR_Scenario_002_cs/HighwayOverhang_18/VISUMatrixSignLights_Mux ==
  MatrixSign_31 : Inport  Tag=inport/MatrixSign_31  PortDimensions=4  SampleTime=1/100  BusOutputAsStruct=on
  MatrixSign_32 : Inport  Tag=inport/MatrixSign_32  Port=2  PortDimensions=4  SampleTime=1/100  BusOutputAsStruct=on
  MuxVisuLights : Mux  Inputs=2
  VISUMatrixSignLights_HighwayOverhang_18 : Outport  Tag=outport/VisuMatrixSignLights  SampleTime=1/100
  wires:
  MuxVisuLights/1 -> VISUMatrixSignLights_HighwayOverhang_18/1
  MatrixSign_31/1 -> MuxVisuLights/1
  MatrixSign_32/1 -> MuxVisuLights/2

== system TSR_Scenario_002_cs/HighwayOverhang_18/VISUMatrixSign_Mux ==
  MatrixSign_31 : Inport
  MatrixSign_32 : Inport  Port=2
  MatrixSign_31_Conversion : DataTypeConversion
  MatrixSign_31_InitialResource : Constant
  MatrixSign_31_Switch : Switch  Criteria=u2 ~= 0
  MatrixSign_32_Conversion : DataTypeConversion
  MatrixSign_32_InitialResource : Constant
  MatrixSign_32_Switch : Switch  Criteria=u2 ~= 0
  SubMuxMatrixSign : Mux  Inputs=2
  MatrixSigns : Outport
  wires:
  SubMuxMatrixSign/1 -> MatrixSigns/1
  MatrixSign_31/1 -> MatrixSign_31_Switch/1, MatrixSign_31_Switch/2
  MatrixSign_31_InitialResource/1 -> MatrixSign_31_Switch/3
  MatrixSign_31_Switch/1 -> MatrixSign_31_Conversion/1
  MatrixSign_31_Conversion/1 -> SubMuxMatrixSign/1
  MatrixSign_32/1 -> MatrixSign_32_Switch/1, MatrixSign_32_Switch/2
  MatrixSign_32_InitialResource/1 -> MatrixSign_32_Switch/3
  MatrixSign_32_Switch/1 -> MatrixSign_32_Conversion/1
  MatrixSign_32_Conversion/1 -> SubMuxMatrixSign/2

== system TSR_Scenario_002_cs/HighwayOverhang_19/VISUMatrixSignLights_Mux ==
  MatrixSign_52 : Inport  Tag=inport/MatrixSign_52  PortDimensions=4  SampleTime=1/100  BusOutputAsStruct=on
  MatrixSign_9 : Inport  Tag=inport/MatrixSign_9  Port=2  PortDimensions=4  SampleTime=1/100  BusOutputAsStruct=on
  MuxVisuLights : Mux  Inputs=2
  VISUMatrixSignLights_HighwayOverhang_19 : Outport  Tag=outport/VisuMatrixSignLights  SampleTime=1/100
  wires:
  MuxVisuLights/1 -> VISUMatrixSignLights_HighwayOverhang_19/1
  MatrixSign_52/1 -> MuxVisuLights/1
  MatrixSign_9/1 -> MuxVisuLights/2

== system TSR_Scenario_002_cs/HighwayOverhang_19/VISUMatrixSign_Mux ==
  MatrixSign_9 : Inport
  MatrixSign_52 : Inport  Port=2
  MatrixSign_52_Conversion : DataTypeConversion
  MatrixSign_52_InitialResource : Constant  Value=8
  MatrixSign_52_Switch : Switch  Criteria=u2 ~= 0
  MatrixSign_9_Conversion : DataTypeConversion
  MatrixSign_9_InitialResource : Constant  Value=8
  MatrixSign_9_Switch : Switch  Criteria=u2 ~= 0
  SubMuxMatrixSign : Mux  Inputs=2
  MatrixSigns : Outport
  wires:
  SubMuxMatrixSign/1 -> MatrixSigns/1
  MatrixSign_9/1 -> MatrixSign_9_Switch/1, MatrixSign_9_Switch/2
  MatrixSign_9_InitialResource/1 -> MatrixSign_9_Switch/3
  MatrixSign_9_Switch/1 -> MatrixSign_9_Conversion/1
  MatrixSign_9_Conversion/1 -> SubMuxMatrixSign/1
  MatrixSign_52/1 -> MatrixSign_52_Switch/1, MatrixSign_52_Switch/2
  MatrixSign_52_InitialResource/1 -> MatrixSign_52_Switch/3
  MatrixSign_52_Switch/1 -> MatrixSign_52_Conversion/1
  MatrixSign_52_Conversion/1 -> SubMuxMatrixSign/2

== system TSR_Scenario_002_cs/HighwayOverhang_2/VISUMatrixSignLights_Mux ==
  MatrixSign_14 : Inport  Tag=inport/MatrixSign_14  PortDimensions=4  SampleTime=1/100  BusOutputAsStruct=on
  MatrixSign_2 : Inport  Tag=inport/MatrixSign_2  Port=2  PortDimensions=4  SampleTime=1/100  BusOutputAsStruct=on
  MuxVisuLights : Mux  Inputs=2
  VISUMatrixSignLights_HighwayOverhang_2 : Outport  Tag=outport/VisuMatrixSignLights  SampleTime=1/100
  wires:
  MuxVisuLights/1 -> VISUMatrixSignLights_HighwayOverhang_2/1
  MatrixSign_14/1 -> MuxVisuLights/1
  MatrixSign_2/1 -> MuxVisuLights/2

== system TSR_Scenario_002_cs/HighwayOverhang_2/VISUMatrixSign_Mux ==
  MatrixSign_14 : Inport
  MatrixSign_2 : Inport  Port=2
  MatrixSign_14_Conversion : DataTypeConversion
  MatrixSign_14_InitialResource : Constant
  MatrixSign_14_Switch : Switch  Criteria=u2 ~= 0
  MatrixSign_2_Conversion : DataTypeConversion
  MatrixSign_2_InitialResource : Constant
  MatrixSign_2_Switch : Switch  Criteria=u2 ~= 0
  SubMuxMatrixSign : Mux  Inputs=2
  MatrixSigns : Outport
  wires:
  SubMuxMatrixSign/1 -> MatrixSigns/1
  MatrixSign_14/1 -> MatrixSign_14_Switch/1, MatrixSign_14_Switch/2
  MatrixSign_14_InitialResource/1 -> MatrixSign_14_Switch/3
  MatrixSign_14_Switch/1 -> MatrixSign_14_Conversion/1
  MatrixSign_14_Conversion/1 -> SubMuxMatrixSign/1
  MatrixSign_2/1 -> MatrixSign_2_Switch/1, MatrixSign_2_Switch/2
  MatrixSign_2_InitialResource/1 -> MatrixSign_2_Switch/3
  MatrixSign_2_Switch/1 -> MatrixSign_2_Conversion/1
  MatrixSign_2_Conversion/1 -> SubMuxMatrixSign/2

== system TSR_Scenario_002_cs/HighwayOverhang_20/VISUMatrixSignLights_Mux ==
  MatrixSign_33 : Inport  Tag=inport/MatrixSign_33  PortDimensions=4  SampleTime=1/100  BusOutputAsStruct=on
  MatrixSign_34 : Inport  Tag=inport/MatrixSign_34  Port=2  PortDimensions=4  SampleTime=1/100  BusOutputAsStruct=on
  MuxVisuLights : Mux  Inputs=2
  VISUMatrixSignLights_HighwayOverhang_20 : Outport  Tag=outport/VisuMatrixSignLights  SampleTime=1/100
  wires:
  MuxVisuLights/1 -> VISUMatrixSignLights_HighwayOverhang_20/1
  MatrixSign_33/1 -> MuxVisuLights/1
  MatrixSign_34/1 -> MuxVisuLights/2

== system TSR_Scenario_002_cs/HighwayOverhang_20/VISUMatrixSign_Mux ==
  MatrixSign_33 : Inport
  MatrixSign_34 : Inport  Port=2
  MatrixSign_33_Conversion : DataTypeConversion
  MatrixSign_33_InitialResource : Constant
  MatrixSign_33_Switch : Switch  Criteria=u2 ~= 0
  MatrixSign_34_Conversion : DataTypeConversion
  MatrixSign_34_InitialResource : Constant
  MatrixSign_34_Switch : Switch  Criteria=u2 ~= 0
  SubMuxMatrixSign : Mux  Inputs=2
  MatrixSigns : Outport
  wires:
  SubMuxMatrixSign/1 -> MatrixSigns/1
  MatrixSign_33/1 -> MatrixSign_33_Switch/1, MatrixSign_33_Switch/2
  MatrixSign_33_InitialResource/1 -> MatrixSign_33_Switch/3
  MatrixSign_33_Switch/1 -> MatrixSign_33_Conversion/1
  MatrixSign_33_Conversion/1 -> SubMuxMatrixSign/1
  MatrixSign_34/1 -> MatrixSign_34_Switch/1, MatrixSign_34_Switch/2
  MatrixSign_34_InitialResource/1 -> MatrixSign_34_Switch/3
  MatrixSign_34_Switch/1 -> MatrixSign_34_Conversion/1
  MatrixSign_34_Conversion/1 -> SubMuxMatrixSign/2

== system TSR_Scenario_002_cs/HighwayOverhang_21/VISUMatrixSignLights_Mux ==
  MatrixSign_11 : Inport  Tag=inport/MatrixSign_11  PortDimensions=4  SampleTime=1/100  BusOutputAsStruct=on
  MatrixSign_53 : Inport  Tag=inport/MatrixSign_53  Port=2  PortDimensions=4  SampleTime=1/100  BusOutputAsStruct=on
  MuxVisuLights : Mux  Inputs=2
  VISUMatrixSignLights_HighwayOverhang_21 : Outport  Tag=outport/VisuMatrixSignLights  SampleTime=1/100
  wires:
  MuxVisuLights/1 -> VISUMatrixSignLights_HighwayOverhang_21/1
  MatrixSign_11/1 -> MuxVisuLights/1
  MatrixSign_53/1 -> MuxVisuLights/2

== system TSR_Scenario_002_cs/HighwayOverhang_21/VISUMatrixSign_Mux ==
  MatrixSign_11 : Inport
  MatrixSign_53 : Inport  Port=2
  MatrixSign_11_Conversion : DataTypeConversion
  MatrixSign_11_InitialResource : Constant  Value=7
  MatrixSign_11_Switch : Switch  Criteria=u2 ~= 0
  MatrixSign_53_Conversion : DataTypeConversion
  MatrixSign_53_InitialResource : Constant  Value=7
  MatrixSign_53_Switch : Switch  Criteria=u2 ~= 0
  SubMuxMatrixSign : Mux  Inputs=2
  MatrixSigns : Outport
  wires:
  SubMuxMatrixSign/1 -> MatrixSigns/1
  MatrixSign_11/1 -> MatrixSign_11_Switch/1, MatrixSign_11_Switch/2
  MatrixSign_11_InitialResource/1 -> MatrixSign_11_Switch/3
  MatrixSign_11_Switch/1 -> MatrixSign_11_Conversion/1
  MatrixSign_11_Conversion/1 -> SubMuxMatrixSign/1
  MatrixSign_53/1 -> MatrixSign_53_Switch/1, MatrixSign_53_Switch/2
  MatrixSign_53_InitialResource/1 -> MatrixSign_53_Switch/3
  MatrixSign_53_Switch/1 -> MatrixSign_53_Conversion/1
  MatrixSign_53_Conversion/1 -> SubMuxMatrixSign/2

== system TSR_Scenario_002_cs/HighwayOverhang_22/VISUMatrixSignLights_Mux ==
  MatrixSign_35 : Inport  Tag=inport/MatrixSign_35  PortDimensions=4  SampleTime=1/100  BusOutputAsStruct=on
  MatrixSign_36 : Inport  Tag=inport/MatrixSign_36  Port=2  PortDimensions=4  SampleTime=1/100  BusOutputAsStruct=on
  MuxVisuLights : Mux  Inputs=2
  VISUMatrixSignLights_HighwayOverhang_22 : Outport  Tag=outport/VisuMatrixSignLights  SampleTime=1/100
  wires:
  MuxVisuLights/1 -> VISUMatrixSignLights_HighwayOverhang_22/1
  MatrixSign_35/1 -> MuxVisuLights/1
  MatrixSign_36/1 -> MuxVisuLights/2

== system TSR_Scenario_002_cs/HighwayOverhang_22/VISUMatrixSign_Mux ==
  MatrixSign_35 : Inport
  MatrixSign_36 : Inport  Port=2
  MatrixSign_35_Conversion : DataTypeConversion
  MatrixSign_35_InitialResource : Constant
  MatrixSign_35_Switch : Switch  Criteria=u2 ~= 0
  MatrixSign_36_Conversion : DataTypeConversion
  MatrixSign_36_InitialResource : Constant
  MatrixSign_36_Switch : Switch  Criteria=u2 ~= 0
  SubMuxMatrixSign : Mux  Inputs=2
  MatrixSigns : Outport
  wires:
  SubMuxMatrixSign/1 -> MatrixSigns/1
  MatrixSign_35/1 -> MatrixSign_35_Switch/1, MatrixSign_35_Switch/2
  MatrixSign_35_InitialResource/1 -> MatrixSign_35_Switch/3
  MatrixSign_35_Switch/1 -> MatrixSign_35_Conversion/1
  MatrixSign_35_Conversion/1 -> SubMuxMatrixSign/1
  MatrixSign_36/1 -> MatrixSign_36_Switch/1, MatrixSign_36_Switch/2
  MatrixSign_36_InitialResource/1 -> MatrixSign_36_Switch/3
  MatrixSign_36_Switch/1 -> MatrixSign_36_Conversion/1
  MatrixSign_36_Conversion/1 -> SubMuxMatrixSign/2

== system TSR_Scenario_002_cs/HighwayOverhang_23/VISUMatrixSignLights_Mux ==
  MatrixSign_13 : Inport  Tag=inport/MatrixSign_13  PortDimensions=4  SampleTime=1/100  BusOutputAsStruct=on
  MatrixSign_54 : Inport  Tag=inport/MatrixSign_54  Port=2  PortDimensions=4  SampleTime=1/100  BusOutputAsStruct=on
  MuxVisuLights : Mux  Inputs=2
  VISUMatrixSignLights_HighwayOverhang_23 : Outport  Tag=outport/VisuMatrixSignLights  SampleTime=1/100
  wires:
  MuxVisuLights/1 -> VISUMatrixSignLights_HighwayOverhang_23/1
  MatrixSign_13/1 -> MuxVisuLights/1
  MatrixSign_54/1 -> MuxVisuLights/2

== system TSR_Scenario_002_cs/HighwayOverhang_23/VISUMatrixSign_Mux ==
  MatrixSign_13 : Inport
  MatrixSign_54 : Inport  Port=2
  MatrixSign_13_Conversion : DataTypeConversion
  MatrixSign_13_InitialResource : Constant  Value=6
  MatrixSign_13_Switch : Switch  Criteria=u2 ~= 0
  MatrixSign_54_Conversion : DataTypeConversion
  MatrixSign_54_InitialResource : Constant  Value=6
  MatrixSign_54_Switch : Switch  Criteria=u2 ~= 0
  SubMuxMatrixSign : Mux  Inputs=2
  MatrixSigns : Outport
  wires:
  SubMuxMatrixSign/1 -> MatrixSigns/1
  MatrixSign_13/1 -> MatrixSign_13_Switch/1, MatrixSign_13_Switch/2
  MatrixSign_13_InitialResource/1 -> MatrixSign_13_Switch/3
  MatrixSign_13_Switch/1 -> MatrixSign_13_Conversion/1
  MatrixSign_13_Conversion/1 -> SubMuxMatrixSign/1
  MatrixSign_54/1 -> MatrixSign_54_Switch/1, MatrixSign_54_Switch/2
  MatrixSign_54_InitialResource/1 -> MatrixSign_54_Switch/3
  MatrixSign_54_Switch/1 -> MatrixSign_54_Conversion/1
  MatrixSign_54_Conversion/1 -> SubMuxMatrixSign/2

== system TSR_Scenario_002_cs/HighwayOverhang_24/VISUMatrixSignLights_Mux ==
  MatrixSign_25 : Inport  Tag=inport/MatrixSign_25  PortDimensions=4  SampleTime=1/100  BusOutputAsStruct=on
  MatrixSign_55 : Inport  Tag=inport/MatrixSign_55  Port=2  PortDimensions=4  SampleTime=1/100  BusOutputAsStruct=on
  MuxVisuLights : Mux  Inputs=2
  VISUMatrixSignLights_HighwayOverhang_24 : Outport  Tag=outport/VisuMatrixSignLights  SampleTime=1/100
  wires:
  MuxVisuLights/1 -> VISUMatrixSignLights_HighwayOverhang_24/1
  MatrixSign_25/1 -> MuxVisuLights/1
  MatrixSign_55/1 -> MuxVisuLights/2

== system TSR_Scenario_002_cs/HighwayOverhang_24/VISUMatrixSign_Mux ==
  MatrixSign_25 : Inport
  MatrixSign_55 : Inport  Port=2
  MatrixSign_25_Conversion : DataTypeConversion
  MatrixSign_25_InitialResource : Constant  Value=5
  MatrixSign_25_Switch : Switch  Criteria=u2 ~= 0
  MatrixSign_55_Conversion : DataTypeConversion
  MatrixSign_55_InitialResource : Constant  Value=5
  MatrixSign_55_Switch : Switch  Criteria=u2 ~= 0
  SubMuxMatrixSign : Mux  Inputs=2
  MatrixSigns : Outport
  wires:
  SubMuxMatrixSign/1 -> MatrixSigns/1
  MatrixSign_25/1 -> MatrixSign_25_Switch/1, MatrixSign_25_Switch/2
  MatrixSign_25_InitialResource/1 -> MatrixSign_25_Switch/3
  MatrixSign_25_Switch/1 -> MatrixSign_25_Conversion/1
  MatrixSign_25_Conversion/1 -> SubMuxMatrixSign/1
  MatrixSign_55/1 -> MatrixSign_55_Switch/1, MatrixSign_55_Switch/2
  MatrixSign_55_InitialResource/1 -> MatrixSign_55_Switch/3
  MatrixSign_55_Switch/1 -> MatrixSign_55_Conversion/1
  MatrixSign_55_Conversion/1 -> SubMuxMatrixSign/2

== system TSR_Scenario_002_cs/HighwayOverhang_25/VISUMatrixSignLights_Mux ==
  MatrixSign_26 : Inport  Tag=inport/MatrixSign_26  PortDimensions=4  SampleTime=1/100  BusOutputAsStruct=on
  MatrixSign_56 : Inport  Tag=inport/MatrixSign_56  Port=2  PortDimensions=4  SampleTime=1/100  BusOutputAsStruct=on
  MuxVisuLights : Mux  Inputs=2
  VISUMatrixSignLights_HighwayOverhang_25 : Outport  Tag=outport/VisuMatrixSignLights  SampleTime=1/100
  wires:
  MuxVisuLights/1 -> VISUMatrixSignLights_HighwayOverhang_25/1
  MatrixSign_26/1 -> MuxVisuLights/1
  MatrixSign_56/1 -> MuxVisuLights/2

== system TSR_Scenario_002_cs/HighwayOverhang_25/VISUMatrixSign_Mux ==
  MatrixSign_26 : Inport
  MatrixSign_56 : Inport  Port=2
  MatrixSign_26_Conversion : DataTypeConversion
  MatrixSign_26_InitialResource : Constant  Value=4
  MatrixSign_26_Switch : Switch  Criteria=u2 ~= 0
  MatrixSign_56_Conversion : DataTypeConversion
  MatrixSign_56_InitialResource : Constant  Value=4
  MatrixSign_56_Switch : Switch  Criteria=u2 ~= 0
  SubMuxMatrixSign : Mux  Inputs=2
  MatrixSigns : Outport
  wires:
  SubMuxMatrixSign/1 -> MatrixSigns/1
  MatrixSign_26/1 -> MatrixSign_26_Switch/1, MatrixSign_26_Switch/2
  MatrixSign_26_InitialResource/1 -> MatrixSign_26_Switch/3
  MatrixSign_26_Switch/1 -> MatrixSign_26_Conversion/1
  MatrixSign_26_Conversion/1 -> SubMuxMatrixSign/1
  MatrixSign_56/1 -> MatrixSign_56_Switch/1, MatrixSign_56_Switch/2
  MatrixSign_56_InitialResource/1 -> MatrixSign_56_Switch/3
  MatrixSign_56_Switch/1 -> MatrixSign_56_Conversion/1
  MatrixSign_56_Conversion/1 -> SubMuxMatrixSign/2

== system TSR_Scenario_002_cs/HighwayOverhang_26/VISUMatrixSignLights_Mux ==
  MatrixSign_37 : Inport  Tag=inport/MatrixSign_37  PortDimensions=4  SampleTime=1/100  BusOutputAsStruct=on
  MatrixSign_38 : Inport  Tag=inport/MatrixSign_38  Port=2  PortDimensions=4  SampleTime=1/100  BusOutputAsStruct=on
  MuxVisuLights : Mux  Inputs=2
  VISUMatrixSignLights_HighwayOverhang_26 : Outport  Tag=outport/VisuMatrixSignLights  SampleTime=1/100
  wires:
  MuxVisuLights/1 -> VISUMatrixSignLights_HighwayOverhang_26/1
  MatrixSign_37/1 -> MuxVisuLights/1
  MatrixSign_38/1 -> MuxVisuLights/2

== system TSR_Scenario_002_cs/HighwayOverhang_26/VISUMatrixSign_Mux ==
  MatrixSign_37 : Inport
  MatrixSign_38 : Inport  Port=2
  MatrixSign_37_Conversion : DataTypeConversion
  MatrixSign_37_InitialResource : Constant
  MatrixSign_37_Switch : Switch  Criteria=u2 ~= 0
  MatrixSign_38_Conversion : DataTypeConversion
  MatrixSign_38_InitialResource : Constant
  MatrixSign_38_Switch : Switch  Criteria=u2 ~= 0
  SubMuxMatrixSign : Mux  Inputs=2
  MatrixSigns : Outport
  wires:
  SubMuxMatrixSign/1 -> MatrixSigns/1
  MatrixSign_37/1 -> MatrixSign_37_Switch/1, MatrixSign_37_Switch/2
  MatrixSign_37_InitialResource/1 -> MatrixSign_37_Switch/3
  MatrixSign_37_Switch/1 -> MatrixSign_37_Conversion/1
  MatrixSign_37_Conversion/1 -> SubMuxMatrixSign/1
  MatrixSign_38/1 -> MatrixSign_38_Switch/1, MatrixSign_38_Switch/2
  MatrixSign_38_InitialResource/1 -> MatrixSign_38_Switch/3
  MatrixSign_38_Switch/1 -> MatrixSign_38_Conversion/1
  MatrixSign_38_Conversion/1 -> SubMuxMatrixSign/2

== system TSR_Scenario_002_cs/HighwayOverhang_27/VISUMatrixSignLights_Mux ==
  MatrixSign_39 : Inport  Tag=inport/MatrixSign_39  PortDimensions=4  SampleTime=1/100  BusOutputAsStruct=on
  MatrixSign_40 : Inport  Tag=inport/MatrixSign_40  Port=2  PortDimensions=4  SampleTime=1/100  BusOutputAsStruct=on
  MuxVisuLights : Mux  Inputs=2
  VISUMatrixSignLights_HighwayOverhang_27 : Outport  Tag=outport/VisuMatrixSignLights  SampleTime=1/100
  wires:
  MuxVisuLights/1 -> VISUMatrixSignLights_HighwayOverhang_27/1
  MatrixSign_39/1 -> MuxVisuLights/1
  MatrixSign_40/1 -> MuxVisuLights/2

== system TSR_Scenario_002_cs/HighwayOverhang_27/VISUMatrixSign_Mux ==
  MatrixSign_39 : Inport
  MatrixSign_40 : Inport  Port=2
  MatrixSign_39_Conversion : DataTypeConversion
  MatrixSign_39_InitialResource : Constant
  MatrixSign_39_Switch : Switch  Criteria=u2 ~= 0
  MatrixSign_40_Conversion : DataTypeConversion
  MatrixSign_40_InitialResource : Constant
  MatrixSign_40_Switch : Switch  Criteria=u2 ~= 0
  SubMuxMatrixSign : Mux  Inputs=2
  MatrixSigns : Outport
  wires:
  SubMuxMatrixSign/1 -> MatrixSigns/1
  MatrixSign_39/1 -> MatrixSign_39_Switch/1, MatrixSign_39_Switch/2
  MatrixSign_39_InitialResource/1 -> MatrixSign_39_Switch/3
  MatrixSign_39_Switch/1 -> MatrixSign_39_Conversion/1
  MatrixSign_39_Conversion/1 -> SubMuxMatrixSign/1
  MatrixSign_40/1 -> MatrixSign_40_Switch/1, MatrixSign_40_Switch/2
  MatrixSign_40_InitialResource/1 -> MatrixSign_40_Switch/3
  MatrixSign_40_Switch/1 -> MatrixSign_40_Conversion/1
  MatrixSign_40_Conversion/1 -> SubMuxMatrixSign/2

== system TSR_Scenario_002_cs/HighwayOverhang_28/VISUMatrixSignLights_Mux ==
  MatrixSign_41 : Inport  Tag=inport/MatrixSign_41  PortDimensions=4  SampleTime=1/100  BusOutputAsStruct=on
  MatrixSign_42 : Inport  Tag=inport/MatrixSign_42  Port=2  PortDimensions=4  SampleTime=1/100  BusOutputAsStruct=on
  MuxVisuLights : Mux  Inputs=2
  VISUMatrixSignLights_HighwayOverhang_28 : Outport  Tag=outport/VisuMatrixSignLights  SampleTime=1/100
  wires:
  MuxVisuLights/1 -> VISUMatrixSignLights_HighwayOverhang_28/1
  MatrixSign_41/1 -> MuxVisuLights/1
  MatrixSign_42/1 -> MuxVisuLights/2

== system TSR_Scenario_002_cs/HighwayOverhang_28/VISUMatrixSign_Mux ==
  MatrixSign_41 : Inport
  MatrixSign_42 : Inport  Port=2
  MatrixSign_41_Conversion : DataTypeConversion
  MatrixSign_41_InitialResource : Constant
  MatrixSign_41_Switch : Switch  Criteria=u2 ~= 0
  MatrixSign_42_Conversion : DataTypeConversion
  MatrixSign_42_InitialResource : Constant
  MatrixSign_42_Switch : Switch  Criteria=u2 ~= 0
  SubMuxMatrixSign : Mux  Inputs=2
  MatrixSigns : Outport
  wires:
  SubMuxMatrixSign/1 -> MatrixSigns/1
  MatrixSign_41/1 -> MatrixSign_41_Switch/1, MatrixSign_41_Switch/2
  MatrixSign_41_InitialResource/1 -> MatrixSign_41_Switch/3
  MatrixSign_41_Switch/1 -> MatrixSign_41_Conversion/1
  MatrixSign_41_Conversion/1 -> SubMuxMatrixSign/1
  MatrixSign_42/1 -> MatrixSign_42_Switch/1, MatrixSign_42_Switch/2
  MatrixSign_42_InitialResource/1 -> MatrixSign_42_Switch/3
  MatrixSign_42_Switch/1 -> MatrixSign_42_Conversion/1
  MatrixSign_42_Conversion/1 -> SubMuxMatrixSign/2

== system TSR_Scenario_002_cs/HighwayOverhang_3/VISUMatrixSignLights_Mux ==
  MatrixSign_12 : Inport  Tag=inport/MatrixSign_12  PortDimensions=4  SampleTime=1/100  BusOutputAsStruct=on
  MatrixSign_50 : Inport  Tag=inport/MatrixSign_50  Port=2  PortDimensions=4  SampleTime=1/100  BusOutputAsStruct=on
  MuxVisuLights : Mux  Inputs=2
  VISUMatrixSignLights_HighwayOverhang_3 : Outport  Tag=outport/VisuMatrixSignLights  SampleTime=1/100
  wires:
  MuxVisuLights/1 -> VISUMatrixSignLights_HighwayOverhang_3/1
  MatrixSign_12/1 -> MuxVisuLights/1
  MatrixSign_50/1 -> MuxVisuLights/2

== system TSR_Scenario_002_cs/HighwayOverhang_3/VISUMatrixSign_Mux ==
  MatrixSign_12 : Inport
  MatrixSign_50 : Inport  Port=2
  MatrixSign_12_Conversion : DataTypeConversion
  MatrixSign_12_InitialResource : Constant  Value=10
  MatrixSign_12_Switch : Switch  Criteria=u2 ~= 0
  MatrixSign_50_Conversion : DataTypeConversion
  MatrixSign_50_InitialResource : Constant  Value=10
  MatrixSign_50_Switch : Switch  Criteria=u2 ~= 0
  SubMuxMatrixSign : Mux  Inputs=2
  MatrixSigns : Outport
  wires:
  SubMuxMatrixSign/1 -> MatrixSigns/1
  MatrixSign_12/1 -> MatrixSign_12_Switch/1, MatrixSign_12_Switch/2
  MatrixSign_12_InitialResource/1 -> MatrixSign_12_Switch/3
  MatrixSign_12_Switch/1 -> MatrixSign_12_Conversion/1
  MatrixSign_12_Conversion/1 -> SubMuxMatrixSign/1
  MatrixSign_50/1 -> MatrixSign_50_Switch/1, MatrixSign_50_Switch/2
  MatrixSign_50_InitialResource/1 -> MatrixSign_50_Switch/3
  MatrixSign_50_Switch/1 -> MatrixSign_50_Conversion/1
  MatrixSign_50_Conversion/1 -> SubMuxMatrixSign/2

== system TSR_Scenario_002_cs/HighwayOverhang_4/VISUMatrixSignLights_Mux ==
  MatrixSign_23 : Inport  Tag=inport/MatrixSign_23  PortDimensions=4  SampleTime=1/100  BusOutputAsStruct=on
  MatrixSign_24 : Inport  Tag=inport/MatrixSign_24  Port=2  PortDimensions=4  SampleTime=1/100  BusOutputAsStruct=on
  MuxVisuLights : Mux  Inputs=2
  VISUMatrixSignLights_HighwayOverhang_4 : Outport  Tag=outport/VisuMatrixSignLights  SampleTime=1/100
  wires:
  MuxVisuLights/1 -> VISUMatrixSignLights_HighwayOverhang_4/1
  MatrixSign_23/1 -> MuxVisuLights/1
  MatrixSign_24/1 -> MuxVisuLights/2

== system TSR_Scenario_002_cs/HighwayOverhang_4/VISUMatrixSign_Mux ==
  MatrixSign_23 : Inport
  MatrixSign_24 : Inport  Port=2
  MatrixSign_23_Conversion : DataTypeConversion
  MatrixSign_23_InitialResource : Constant
  MatrixSign_23_Switch : Switch  Criteria=u2 ~= 0
  MatrixSign_24_Conversion : DataTypeConversion
  MatrixSign_24_InitialResource : Constant
  MatrixSign_24_Switch : Switch  Criteria=u2 ~= 0
  SubMuxMatrixSign : Mux  Inputs=2
  MatrixSigns : Outport
  wires:
  SubMuxMatrixSign/1 -> MatrixSigns/1
  MatrixSign_23/1 -> MatrixSign_23_Switch/1, MatrixSign_23_Switch/2
  MatrixSign_23_InitialResource/1 -> MatrixSign_23_Switch/3
  MatrixSign_23_Switch/1 -> MatrixSign_23_Conversion/1
  MatrixSign_23_Conversion/1 -> SubMuxMatrixSign/1
  MatrixSign_24/1 -> MatrixSign_24_Switch/1, MatrixSign_24_Switch/2
  MatrixSign_24_InitialResource/1 -> MatrixSign_24_Switch/3
  MatrixSign_24_Switch/1 -> MatrixSign_24_Conversion/1
  MatrixSign_24_Conversion/1 -> SubMuxMatrixSign/2

== system TSR_Scenario_002_cs/HighwayOverhang_5/VISUMatrixSignLights_Mux ==
  MatrixSign_48 : Inport  Tag=inport/MatrixSign_48  PortDimensions=4  SampleTime=1/100  BusOutputAsStruct=on
  MatrixSign_8 : Inport  Tag=inport/MatrixSign_8  Port=2  PortDimensions=4  SampleTime=1/100  BusOutputAsStruct=on
  MuxVisuLights : Mux  Inputs=2
  VISUMatrixSignLights_HighwayOverhang_5 : Outport  Tag=outport/VisuMatrixSignLights  SampleTime=1/100
  wires:
  MuxVisuLights/1 -> VISUMatrixSignLights_HighwayOverhang_5/1
  MatrixSign_48/1 -> MuxVisuLights/1
  MatrixSign_8/1 -> MuxVisuLights/2

== system TSR_Scenario_002_cs/HighwayOverhang_5/VISUMatrixSign_Mux ==
  MatrixSign_8 : Inport
  MatrixSign_48 : Inport  Port=2
  MatrixSign_48_Conversion : DataTypeConversion
  MatrixSign_48_InitialResource : Constant  Value=12
  MatrixSign_48_Switch : Switch  Criteria=u2 ~= 0
  MatrixSign_8_Conversion : DataTypeConversion
  MatrixSign_8_InitialResource : Constant  Value=12
  MatrixSign_8_Switch : Switch  Criteria=u2 ~= 0
  SubMuxMatrixSign : Mux  Inputs=2
  MatrixSigns : Outport
  wires:
  SubMuxMatrixSign/1 -> MatrixSigns/1
  MatrixSign_8/1 -> MatrixSign_8_Switch/1, MatrixSign_8_Switch/2
  MatrixSign_8_InitialResource/1 -> MatrixSign_8_Switch/3
  MatrixSign_8_Switch/1 -> MatrixSign_8_Conversion/1
  MatrixSign_8_Conversion/1 -> SubMuxMatrixSign/1
  MatrixSign_48/1 -> MatrixSign_48_Switch/1, MatrixSign_48_Switch/2
  MatrixSign_48_InitialResource/1 -> MatrixSign_48_Switch/3
  MatrixSign_48_Switch/1 -> MatrixSign_48_Conversion/1
  MatrixSign_48_Conversion/1 -> SubMuxMatrixSign/2

== system TSR_Scenario_002_cs/HighwayOverhang_6/VISUMatrixSignLights_Mux ==
  MatrixSign_19 : Inport  Tag=inport/MatrixSign_19  PortDimensions=4  SampleTime=1/100  BusOutputAsStruct=on
  MatrixSign_20 : Inport  Tag=inport/MatrixSign_20  Port=2  PortDimensions=4  SampleTime=1/100  BusOutputAsStruct=on
  MuxVisuLights : Mux  Inputs=2
  VISUMatrixSignLights_HighwayOverhang_6 : Outport  Tag=outport/VisuMatrixSignLights  SampleTime=1/100
  wires:
  MuxVisuLights/1 -> VISUMatrixSignLights_HighwayOverhang_6/1
  MatrixSign_19/1 -> MuxVisuLights/1
  MatrixSign_20/1 -> MuxVisuLights/2
